simulink library "quat_matrix"  (R2019b)
settings: Solver=VariableStepAuto  StartTime=0.0  StopTime=10.0  RelTol=1e-3  EnableMultiTasking=on
settings Model: Creator=rivolta  LastModifiedBy=AurelianoRivolta
settings DataIOCC: LimitDataPoints=on  ReturnWorkspaceOutputs=off
settings OptimizationCC: LifeSpan=inf
settings DebuggingCC: AllowSymbolicDim=off  SFUnexpectedBacktrackingDiag=warning  SFNoUnconditionalDefaultTransitionDiag=warning  SFExecutionAtInitializationDiag=none  ArithmeticOperatorsInVariantConditions=warning
settings ModelReferenceCC: PropagateSignalLabelsOutOfModel=off
settings SFSimCC: SimUseLocalCustomCode=off  CustomCodeUndefinedFunction=UseInterfaceOnly
settings RTWCC: RTWUseLocalCustomCode=off
settings CodeAppCC: StateflowObjectComments=on
settings GRTTargetCC: TargetLangStandard=C89/C90 (ANSI)
settings ConfigComp: CovMetricSettings=dw  CovHtmlReporting=on  CovSaveCumulativeToWorkspaceVar=on  CovSaveSingleToWorkspaceVar=on  CovExternalEMLEnable=off

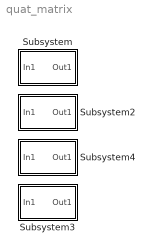
== system quat_matrix ==
  Subsystem : Subsystem
      mask help: crossqm
      mask Help:
      | % Author: Aureliano Rivolta
      | % e-mail: aureliano.rivolta@polimi.it
      | % year: 2016
      | % private use only
      mask Display:
      | port_label('input',1,'\bf q','interpreter','tex')
      | port_label('output',1,'[\bf{q} \otimes -]','interpreter','tex')
  Subsystem2 : Subsystem
      mask help: crossqp
      mask Help:
      | % Author: Aureliano Rivolta
      | % e-mail: aureliano.rivolta@polimi.it
      | % year: 2016
      | % private use only
      mask Display:
      | port_label('input',1,'\bf q','interpreter','tex')
      | port_label('output',1,'[\bf{q} \otimes +]','interpreter','tex')
  Subsystem3 : Subsystem
      mask help: crossqpt
      mask Help:
      | % Author: Aureliano Rivolta
      | % e-mail: aureliano.rivolta@polimi.it
      | % year: 2016
      | % private use only
      mask Display:
      | port_label('input',1,'\bf q','interpreter','tex')
      | port_label('output',1,'[\bf{q} \otimes +^T]','interpreter','tex')
  Subsystem4 : Subsystem
      mask help: crossqmt
      mask Help:
      | % Author: Aureliano Rivolta
      | % e-mail: aureliano.rivolta@polimi.it
      | % year: 2016
      | % private use only
      mask Display:
      | port_label('input',1,'\bf q','interpreter','tex')
      | port_label('output',1,'[\bf{q} \otimes - ^T]','interpreter','tex')

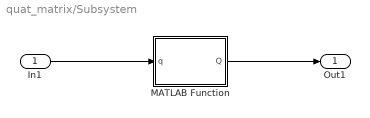
== system quat_matrix/Subsystem ==
  In1 : Inport
  MATLAB Function : MATLAB Function  TreatAsAtomicUnit=on
  Out1 : Outport
  wires:
  MATLAB Function/1(Q) -> Out1/1
  In1/1 -> MATLAB Function/1(q)

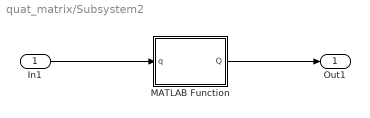
== system quat_matrix/Subsystem2 ==
  In1 : Inport
  MATLAB Function : MATLAB Function  TreatAsAtomicUnit=on
  Out1 : Outport
  wires:
  MATLAB Function/1(Q) -> Out1/1
  In1/1 -> MATLAB Function/1(q)

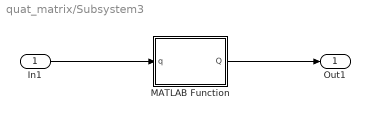
== system quat_matrix/Subsystem3 ==
  In1 : Inport
  MATLAB Function : MATLAB Function  TreatAsAtomicUnit=on
  Out1 : Outport
  wires:
  MATLAB Function/1(Q) -> Out1/1
  In1/1 -> MATLAB Function/1(q)

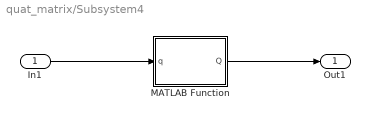
== system quat_matrix/Subsystem4 ==
  In1 : Inport
  MATLAB Function : MATLAB Function  TreatAsAtomicUnit=on
  Out1 : Outport
  wires:
  MATLAB Function/1(Q) -> Out1/1
  In1/1 -> MATLAB Function/1(q)

== matlab function quat_matrix/Subsystem/MATLAB Function ==
  data: q input; Q output
function Q = fcn(q)
%#codegen

Q = crossqm(q);

== matlab function quat_matrix/Subsystem2/MATLAB Function ==
  data: q input; Q output
function Q = fcn(q)
%#codegen

Q = crossqp(q);

== matlab function quat_matrix/Subsystem3/MATLAB Function ==
  data: q input; Q output
function Q = fcn(q)
%#codegen

Q = crossqpt(q);

== matlab function quat_matrix/Subsystem4/MATLAB Function ==
  data: q input; Q output
function Q = fcn(q)
%#codegen

Q = crossqmt(q);
